simulink model "Tanksim"  (R2025b)
settings: Solver=FixedStepAuto  StartTime=0.0  StopTime=1635  FixedStep=1  RelTol=1e-3
values from neighbouring files (symbols this model uses):
  a = q0/sqrt(2*g*h_10)    [Tanktest.m]    (also in Tanktest.mat = 0.278710327833)
  A = Tvarsnitssarea    (= 32.1699087728)    [Tanktest.m]    (also in Tanktest.mat)
  alfa = a/(2*A)*sqrt(2*g/(h_10))    [Tanktest.m]    (also in Tanktest.mat = 0.0678733031674)
  g = 982    [Tanktest.m]    (also in Tanktest.mat)
  K12 = 1    [Tanktest.m]    (also in Tanktest.mat)
  P = polyfit(M,H,1)    [Tanktest.m]    (also in Tanktest.mat = [1.78625593595 -0.0624313169737])
  qDq = (q_val-q0)/(V_val-u0)    [Tanktest.m]    (also in Tanktest.mat = 5.81123494738)
  T = 2*Tvarsnitssarea/a*sqrt(h_10/(2*g))    [Tanktest.m]    (also in Tanktest.mat = 14.7333333333)
settings Model: Creator=thelig-3  LastModifiedBy=thelig-3

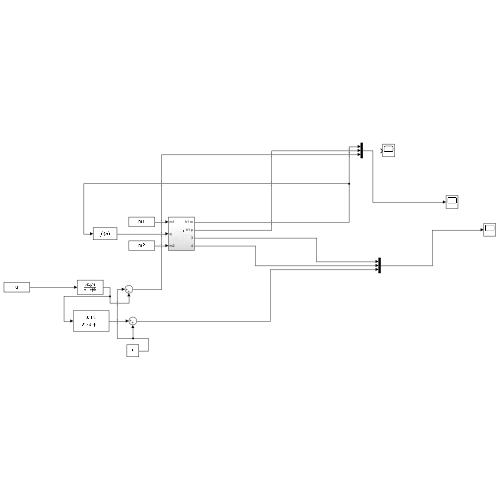
[thumbnail: Simulink's stored preview of the top-level diagram]
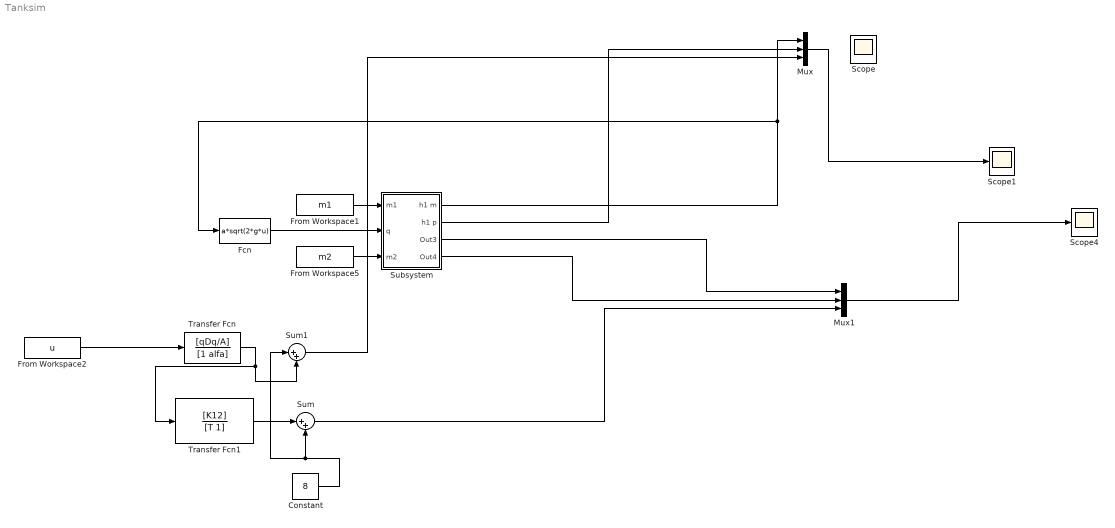
== system Tanksim ==
  Constant : Constant  Value=8
  Fcn : Fcn  Expr=a*sqrt(2*g*u)
  From Workspace1 : FromWorkspace  VariableName=m1
  From Workspace2 : FromWorkspace  VariableName=u
  From Workspace5 : FromWorkspace  VariableName=m2
  Mux : Mux  Inputs=3
  Mux1 : Mux  Inputs=3
  Scope : Scope
      settings: ActiveDisplayYMinimum=-3.3137371616583255  ActiveDisplayYMaximum=14.01114590158128
  Scope1 : Scope
      settings: Title=Övre tankens vatten nivå mot tiden>  ActiveDisplayYMinimum=-6.310822026424729  ActiveDisplayYMaximum=22.679377505797572  YLabel=h_1
  Scope4 : Scope
      settings: Title=Undre tankens vatten nivå mot tiden>  ActiveDisplayYMinimum=-6.310822026424729  ActiveDisplayYMaximum=22.679377505797572  YLabel=h_2  DataLoggingVariableName=ScopeData4
  Subsystem : Subsystem
  Sum : Sum  Inputs=|++
  Sum1 : Sum  Inputs=|++
  Transfer Fcn : TransferFcn  Numerator=[qDq/A]  Denominator=[1 alfa]
  Transfer Fcn1 : TransferFcn  Numerator=[K12]  Denominator=[T 1]
  wires:
  Mux1/1 -> Scope4/1
  Subsystem/1(h1 m) -> Mux/1, Fcn/1
  From Workspace1/1 -> Subsystem/1(m1)
  Fcn/1 -> Subsystem/2(q)
  Subsystem/2(h1 p) -> Mux/2
  Subsystem/3(Out3) -> Mux1/1
  Subsystem/4(Out4) -> Mux1/2
  From Workspace5/1 -> Subsystem/3(m2)
  From Workspace2/1 -> Transfer Fcn/1
  Constant/1 -> Sum1/1, Sum/2
  Transfer Fcn1/1 -> Sum/1
  Transfer Fcn/1 -> Transfer Fcn1/1, Sum1/2
  Sum1/1 -> Mux/3
  Sum/1 -> Mux1/3
  Mux/1 -> Scope1/1

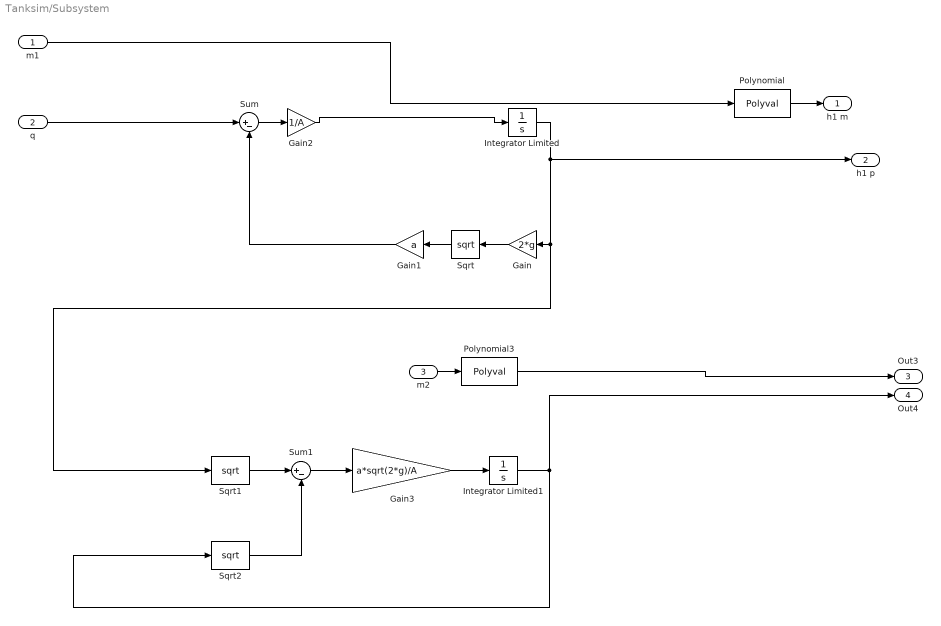
== system Tanksim/Subsystem ==
  m1 : Inport
  q : Inport  Port=2
  m2 : Inport  Port=3
  Gain : Gain  Gain=2*g
  Gain1 : Gain  Gain=a
  Gain2 : Gain  Gain=1/A
  Gain3 : Gain  Gain=a*sqrt(2*g)/A
  Integrator Limited : Integrator  LimitOutput=on  LowerSaturationLimit=0
  Integrator Limited1 : Integrator  LimitOutput=on  LowerSaturationLimit=0
  Polynomial : Polyval  Coefs=P
  Polynomial3 : Polyval  Coefs=P
  Sqrt : Sqrt
  Sqrt1 : Sqrt
  Sqrt2 : Sqrt
  Sum : Sum  Inputs=|+-
  Sum1 : Sum  Inputs=|+-
  h1 m : Outport
  h1 p : Outport  Port=2
  Out3 : Outport  Port=3
  Out4 : Outport  Port=4
  wires:
  Polynomial3/1 -> Out3/1
  Integrator Limited/1 -> h1 p/1, Sqrt1/1, Gain/1
  Gain2/1 -> Integrator Limited/1
  q/1 -> Sum/1
  Sum/1 -> Gain2/1
  Gain/1 -> Sqrt/1
  Sqrt/1 -> Gain1/1
  Sqrt1/1 -> Sum1/1
  Gain1/1 -> Sum/2
  Gain3/1 -> Integrator Limited1/1
  Integrator Limited1/1 -> Out4/1, Sqrt2/1
  Sum1/1 -> Gain3/1
  Sqrt2/1 -> Sum1/2
  m1/1 -> Polynomial/1
  Polynomial/1 -> h1 m/1
  m2/1 -> Polynomial3/1
